simulink library "Banshee_SEL751_Woodward_lib"  (Simulink 8.1)
settings: Solver=ode45  StartTime=0.0  StopTime=10.0  RelTol=1e-3
undefined symbols (not defined in the file): fdesignblkfcn, gcbh
libraries: rtio_opalrt_common x13, rtio_opalrt_op5142ex1 x12, simulink x10, simulink_extras x8
(part 2 of 2)

== system Banshee_SEL751_Woodward_lib/Banshee_HWCtrl_IOs/Woodward Outputs - Diesel - Gen2/Woodward Primary Inputs - Gen2/Lowpass Filter2 ==
  In : Inport
  Generated Filter Block : DiscreteFir  Tag=BlockMethodSubSystem  Coefficients=[0.0069552863617617106 0.014587901014631248 -0.0057896483056441538 -0.056861876528372622 -0.059476680260783142 0.076118200884714562 0.29579154768342669 0.40638624201187618 0.29579154768342669 0.076118200884714562 -0.059476680260783142 -0.056861876528372622 -0.0057896483056441538 0.014587901014631248 0.0069552863617617106]  InputProcessing=Columns as channels (frame based)
  Out : Outport
  wires:
  Generated Filter Block/1 -> Out/1
  In/1 -> Generated Filter Block/1

== system Banshee_SEL751_Woodward_lib/Banshee_HWCtrl_IOs/Woodward Outputs - Diesel - Gen2/Woodward Primary Inputs - Gen2/Lowpass Filter3 ==
  In : Inport
  Generated Filter Block : DiscreteFir  Tag=BlockMethodSubSystem  Coefficients=[0.0069552863617617106 0.014587901014631248 -0.0057896483056441538 -0.056861876528372622 -0.059476680260783142 0.076118200884714562 0.29579154768342669 0.40638624201187618 0.29579154768342669 0.076118200884714562 -0.059476680260783142 -0.056861876528372622 -0.0057896483056441538 0.014587901014631248 0.0069552863617617106]  InputProcessing=Columns as channels (frame based)
  Out : Outport
  wires:
  Generated Filter Block/1 -> Out/1
  In/1 -> Generated Filter Block/1

== system Banshee_SEL751_Woodward_lib/Banshee_HWCtrl_IOs/Woodward Outputs - NGCHP - Gen1/DIO - Gr3/Conditioning ==
  In1 : Inport
  Bus Creator : BusCreator  Inputs=8
  Demux : Demux  Outputs=8
  Out1 : Outport
  wires:
  In1/1 -> Demux/1
  Bus Creator/1 -> Out1/1  "DI_CH00-07"
  Demux/8 -> Bus Creator/8  "Gen1_Alarm_CF"
  Demux/7 -> Bus Creator/7  "Gen1_Alarm_AB"
  Demux/6 -> Bus Creator/6  "Gen1_Open_MCB"
  Demux/5 -> Bus Creator/5  "Gen1_Close_MCB"
  Demux/4 -> Bus Creator/4  "Gen1_Open_GCB"
  Demux/3 -> Bus Creator/3  "Gen1_Close_GCB"
  Demux/2 -> Bus Creator/2  "Gen1_Fuel"
  Demux/1 -> Bus Creator/1  "Gen1_Starter"

== system Banshee_SEL751_Woodward_lib/Banshee_HWCtrl_IOs/Woodward Outputs - NGCHP - Gen1/Woodward Primary Inputs - Gen1/Lowpass Filter ==
  In : Inport
  Generated Filter Block : DiscreteFir  Tag=BlockMethodSubSystem  Coefficients=[0.0069552863617617106 0.014587901014631248 -0.0057896483056441538 -0.056861876528372622 -0.059476680260783142 0.076118200884714562 0.29579154768342669 0.40638624201187618 0.29579154768342669 0.076118200884714562 -0.059476680260783142 -0.056861876528372622 -0.0057896483056441538 0.014587901014631248 0.0069552863617617106]  InputProcessing=Columns as channels (frame based)
  Out : Outport
  wires:
  Generated Filter Block/1 -> Out/1
  In/1 -> Generated Filter Block/1

== system Banshee_SEL751_Woodward_lib/Banshee_HWCtrl_IOs/Woodward Outputs - NGCHP - Gen1/Woodward Primary Inputs - Gen1/Lowpass Filter1 ==
  In : Inport
  Generated Filter Block : DiscreteFir  Tag=BlockMethodSubSystem  Coefficients=[0.0069552863617617106 0.014587901014631248 -0.0057896483056441538 -0.056861876528372622 -0.059476680260783142 0.076118200884714562 0.29579154768342669 0.40638624201187618 0.29579154768342669 0.076118200884714562 -0.059476680260783142 -0.056861876528372622 -0.0057896483056441538 0.014587901014631248 0.0069552863617617106]  InputProcessing=Columns as channels (frame based)
  Out : Outport
  wires:
  Generated Filter Block/1 -> Out/1
  In/1 -> Generated Filter Block/1
